simulink model "Simulation_control"  (R2024a)
settings: Solver=ode4  StartTime=0.0  StopTime=105  FixedStep=0.01  RelTol=1e-3
InitFcn:
  | SimInit
values from neighbouring files (symbols this model uses):
  A_mdl = [A11 0 0 ... (first row only)    [SimInit.m]
  B_mdl = l*Kvt/(r*R) * [0 sqrt(3)/(2*M), -sqrt(3)/(2*M) ... (first row only)    [SimInit.m]
  k1_smc = diag([0.7206586704988028 0.846888480151037 0.848909652523])    [SimInit.m]
  k2_smc = diag([1.3 1.32370704517714 1.1]) * k1_smc    [SimInit.m]
  K_mdl = [-Cv/M 0 0 ... (first row only)    [SimInit.m]
  Q_smc = 0.1*diag([1, 1, 1])    [SimInit.m]
settings Model: Creator=irfan  LastModifiedBy=irfan
settings DataIOCC: LimitDataPoints=on  MaxDataPoints=1

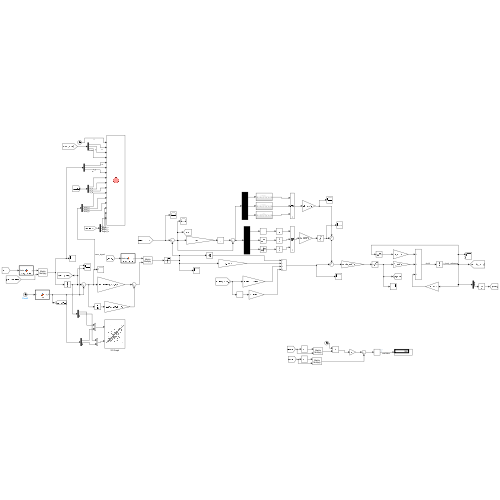
[thumbnail: Simulink's stored preview of the top-level diagram]
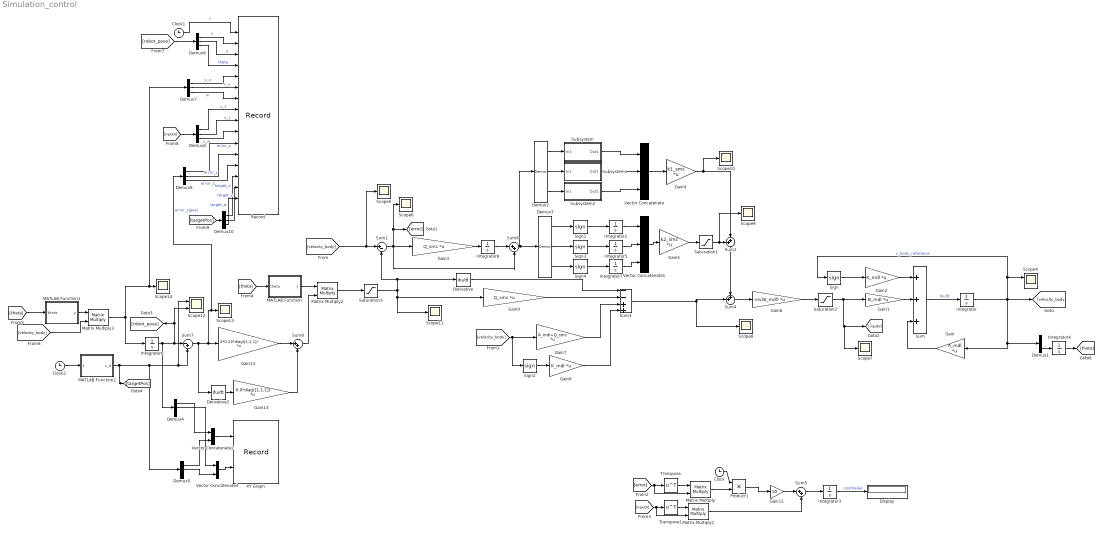
== system Simulation_control ==
  Clock : Clock
  Clock1 : Clock
  Clock2 : Clock
  Demux{1..10} (10 alike) : Demux  Outputs=3
  Derivative : Derivative
  Derivative2 : Derivative
  Display : Display
  Gain : Gain  Gain=A_mdl  Multiplication=Matrix(K*u)
  Gain1 : Gain  Gain=B_mdl  Multiplication=Matrix(K*u)
  Gain11 : Gain  Gain=10
  Gain13 : Gain  Gain=4*0.23*diag([1,1,1])  Multiplication=Matrix(K*u)
  Gain14 : Gain  Gain=0.9*diag([1,1,1])  Multiplication=Matrix(K*u)
  Gain2 : Gain  Gain=K_mdl  Multiplication=Matrix(K*u)
  Gain3 : Gain  Gain=Q_smc  Multiplication=Matrix(K*u)
  Gain4 : Gain  Gain=k1_smc  Multiplication=Matrix(K*u)
  Gain5 : Gain  Gain=k2_smc  Multiplication=Matrix(K*u)
  Gain6 : Gain  Gain=-inv(B_mdl)  Multiplication=Matrix(K*u)
  Gain7 : Gain  Gain=A_mdl+Q_smc  Multiplication=Matrix(K*u)
  Gain8 : Gain  Gain=K_mdl  Multiplication=Matrix(K*u)
  Gain9 : Gain  Gain=Q_smc  Multiplication=Matrix(K*u)
  Integrator{,2..5,7..8} (7 alike) : Integrator
  Integrator6 : Integrator  InitialCondition=[2;-1;0]
  MATLAB Function : MATLAB Function  TreatAsAtomicUnit=on
  MATLAB Function1 : MATLAB Function  TreatAsAtomicUnit=on
  MATLAB Function2 : MATLAB Function  TreatAsAtomicUnit=on
  Matrix Multiply{,1..3} (4 alike) : Product  Multiplication=Matrix(*)
  Product1 : Product
  Record : Record  Filename=result_10kg.mat  RecordToFile=on  FileSettingsInternal="{\"entries\":[{\"content\":{\"excelSettings\":{\"content\":{},\"type\":\"Streamout.ExcelSettings\"}},\"type\":\"Streamout.FileSettingStorage\",\"uuid\":\"\"}],\"packageUris\":[\"http:\\/\\/schema.mathworks.com\\/mf0\\/streamout_blocks\\/R2020a\"],\"version\":\"1.0\"}"  SignalsInternal="{\"entries\":[{\"content\":{\"signals\":[{\"content\":{\"blockPath\":[],\"dimensions\":[1],\"domain\":\"\",\"lineColor\":\"#64d413\",\"lineWidth\":2,\"plots\":[ 1 ],\"port\":1,\"sid\":[\"\"],\"signalID\":1,\"signalName\":\"t\"},\"type\":\"RecordBlkView.Signal\",\"uuid\":\"\"},{\"content\":{\"blockPath\":[],\"dimensions\":[1,1],\"domain\":\"\",\"lineColor\":\"#ff13a6\",\"lineWidth\":2,\"plots\":[ 1 ],\"port\":2,\"sid\":[\"\"],\"signalID\":2,\"signalName\":\"x\"},\"type\":\"RecordBlkView.Signal\",\"uuid\":\"\"},{\"content\":{\"blockPath\":[],\"dimensions\":[1,1],\"domain\":\"\",\"lineColor\":\"#fe330a\",\"lineWidth\":2,\"plots\":[ 1 ],\"port\":3,\"sid\":[\"\"],\"signalID\":3,\"signalName\":\"y\"},\"type\":\"RecordBlkView.Signal\",\"uuid\":\"\"},{\"content\":{\"blockPath\":[],\"dimensions\":[1,1],\"domain\":\"\",\"lineColor\":\"#22b573\",\"lineWidth\":2,\"plots\":[ 1 ],\"port\":4,\"sid\":[\"\"],\"signalID\":4,\"signalName\":\"theta\"},\"type\":\"RecordBlkView.Signal\",\"uuid\":\"\"},{\"content\":{\"blockPath\":[],\"dimensions\":[1,1],\"domain\":\"\",\"lineColor\":\"#0072bd\",\"lineWidth\":2,\"plots\":[ 1 ],\"port\":5,\"sid\":[\"\"],\"signalID\":5,\"signalName\":\"v_x\"},\"type\":\"RecordBlkView.Signal\",\"uuid\":\"\"},{\"content\":{\"blockPath\":[],\"dimensions\":[1,1],\"domain\":\"\",\"lineColor\":\"#d95319\",\"lineWidth\":2,\"plots\":[ 1 ],\"port\":6,\"sid\":[\"\"],\"signalID\":6,\"signalName\":\"v_y\"},\"type\":\"RecordBlkView.Signal\",\"uuid\":\"\"},{\"content\":{\"blockPath\":[],\"dimensions\":[1,1],\"domain\":\"\",\"lineColor\":\"#edb120\",\"lineWidth\":2,\"plots\":[ 1 ],\"port\":7,\"sid\":[\"\"],\"signalID\":7,\"signalName\":\"w\"},\"type\":\"RecordBlkView.Signal\",\"uuid\":\"\"},{\"content\":{\"blockPath\":[],\"dimensions\":[1,1],\"domain\":\"\",\"lineColor\":\"#a2142f\",\"lineWidth\":2,\"plots\":[ 1 ],\"port\":8,\"sid\":[\"\"],\"signalID\":8,\"signalName\":\"u_x\"},\"type\":\"RecordBlkView.Signal\",\"uuid\":\"\"},{\"content\":{\"blockPath\":[],\"dimensions\":[1,1],\"domain\":\"\",\"lineColor\":\"#139fff\",\"lineWidth\":2,\"plots\":[ 1 ],\"port\":9,\"sid\":[\"\"],\"signalID\":9,\"signalName\":\"u_y\"},\"type\":\"RecordBlkView.Signal\",\"uuid\":\"\"},{\"content\":{\"blockPath\":[],\"dimensions\":[1,1],\"domain\":\"\",\"lineColor\":\"#ff6929\",\"lineWidth\":2,\"plots\":[ 1 ],\"port\":10,\"sid\":[\"\"],\"signalID\":10,\"signalName\":\"u_w\"},\"type\":\"RecordBlkView.Signal\",\"uuid\":\"\"},{\"content\":{\"blockPath\":[],\"dimensions\":[1,1],\"domain\":\"\",\"lineColor\":\"#b746ff\",\"lineWidth\":2,\"plots\":[ 1 ],\"port\":11,\"sid\":[\"\"],\"signalID\":11,\"signalName\":\"error_x\"},\"type\":\"RecordBlkView.Signal\",\"uuid\":\"\"},{\"content\":{\"blockPath\":[],\"dimensions\":[1,1],\"domain\":\"\",\"lineColor\":\"#64d413\",\"lineWidth\":2,\"plots\":[ 1 ],\"port\":12,\"sid\":[\"\"],\"signalID\":12,\"signalName\":\"error_y\"},\"type\":\"RecordBlkView.Signal\",\"uuid\":\"\"},{\"content\":{\"blockPath\":[],\"dimensions\":[1,1],\"domain\":\"\",\"lineColor\":\"#ff13a6\",\"lineWidth\":2,\"plots\":[ 1 ],\"port\":13,\"sid\":[\"\"],\"signalID\":13,\"signalName\":\"error_z\"},\"type\":\"RecordBlkView.Signal\",\"uuid\":\"\"},{\"content\":{\"blockPath\":[],\"dimensions\":[1,1],\"domain\":\"\",\"lineColor\":\"#77ac30\",\"lineWidth\":2,\"plots\":[ 1 ],\"port\":14,\"sid\":[\"\"],\"signalID\":14,\"signalName\":\"target_x\"},\"type\":\"RecordBlkView.Signal\",\"uuid\":\"\"},{\"content\":{\"blockPath\":[],\"dimensions\":[1,1],\"domain\":\"\",\"lineColor\":\"#4dbeee\",\"lineWidth\":2,\"plots\":[ 1 ],\"port\":15,\"sid\":[\"\"],\"signalID\":15,\"signalName\":\"target_y\"},\"type\":\"RecordBlkView.Signal\",\"uuid\":\"\"},{\"content\":{\"blockPath\":[],\"dimensions\":[1,1],\"domain\":\"\",\"lineColor\":\"#a2142f\",\"lineWidth\":2,\"plots\":[ 1 ],\"port\":16,\"sid\":[\"\"],\"signalID\":16,\"signalName\":\"target_w\"},\"type\":\"RecordBlkView.Signal\",\"uuid\":\"\"}]},\"type\":\"RecordBlkView.InputSignals\",\"uuid\":\"\"}],\"packageUris\":[\"http:\\/\\/schema.mathworks.com\\/mf0\\/streamout_blocks\\/R2020a\"],\"version\":\"1.0\"}"  VisualizationBindings="{\"sparklinesplugin\":{\"info\":[{\"bindingParametersList\":[],\"subplotID\":1}]}}"
  Saturation1 : Saturate  UpperLimit=12  LowerLimit=-12
  Saturation2 : Saturate  UpperLimit=6  LowerLimit=-6
  Saturation3 : Saturate  UpperLimit=[2.3;2.3;28]  LowerLimit=-[2.3;2.3;28]
  Scope{5..11,13..14} (9 alike) : Scope
  Scope12 : Scope  NumInputPorts=2
  Scope4 : Scope  NumInputPorts=2
  Sign{,1..4} (5 alike) : Signum
  Subsystem : Subsystem
  Subsystem1 : Subsystem
  Subsystem2 : Subsystem
  Sum : Sum  Inputs=+++
  Sum1 : Sum  Inputs=|+-
  Sum2 : Sum  Inputs=++|
  Sum3 : Sum  Inputs=--++
  Sum4 : Sum  Inputs=++|
  Sum5 : Sum  Inputs=|++
  Sum6 : Sum  Inputs=|++
  Sum7 : Sum  Inputs=|-+
  Sum8 : Sum  Inputs=|++
  Transpose : Math  Operator=transpose
  Transpose1 : Math  Operator=transpose
  Vector Concatenate : Concatenate  NumInputs=3  Mode=Multidimensional array
  Vector Concatenate1 : Concatenate  NumInputs=3  Mode=Multidimensional array
  Vector Concatenate2 : Concatenate  Mode=Multidimensional array
  Vector Concatenate3 : Concatenate  Mode=Multidimensional array
  XY Graph : Record  Filename=recording.mat  RecordToFile=on  FileSettingsInternal="{\"entries\":[{\"content\":{\"excelSettings\":{\"content\":{},\"type\":\"Streamout.ExcelSettings\"}},\"type\":\"Streamout.FileSettingStorage\",\"uuid\":\"\"}],\"packageUris\":[\"http:\\/\\/schema.mathworks.com\\/mf0\\/streamout_blocks\\/R2020a\"],\"version\":\"1.0\"}"  Layout=[1 1]  SignalsInternal="{\"entries\":[{\"content\":{\"signals\":[{\"content\":{\"blockPath\":[],\"dimensions\":[2,1],\"domain\":\"\",\"hasChildren\":true,\"lineColor\":\"#ff6929\",\"lineWidth\":2,\"port\":1,\"sid\":[\"\"],\"signalID\":1,\"signalName\":\"Vector\\nConcatenate2\"},\"type\":\"RecordBlkView.Signal\",\"uuid\":\"\"},{\"content\":{\"blockPath\":[],\"channel\":[1,1],\"dimensions\":[2,1],\"domain\":\"\",\"lineColor\":\"#edb120\",\"lineWidth\":2,\"parentID\":1,\"plots\":[ 1 ],\"port\":1,\"sid\":[\"\"],\"signalID\":2,\"signalName\":\"Vector\\nConcatenate2\"},\"type\":\"RecordBlkView.Signal\",\"uuid\":\"\"},{\"content\":{\"blockPath\":[],\"dimensions\":[2,1],\"domain\":\"\",\"hasChildren\":true,\"lineColor\":\"#64d413\",\"lineWidth\":2,\"port\":2,\"sid\":[\"\"],\"signalID\":3,\"signalName\":\"Vector\\nConcatenate3\"},\"type\":\"RecordBlkView.Signal\",\"uuid\":\"\"},{\"content\":{\"blockPath\":[],\"channel\":[1,1],\"dimensions\":[2,1],\"domain\":\"\",\"lineColor\":\"#77ac30\",\"lineWidth\":2,\"parentID\":3,\"plots\":[ 1 ],\"port\":2,\"sid\":[\"\"],\"signalID\":4,\"signalName\":\"Vector\\nConcatenate3\"},\"type\":\"RecordBlkView.Signal\",\"uuid\":\"\"},{\"content\":{\"blockPath\":[],\"channel\":[2,1],\"dimensions\":[2,1],\"domain\":\"\",\"lineColor\":\"#4dbeee\",\"lineWidth\":2,\"parentID\":1,\"plots\":[ 1 ],\"port\":1,\"sid\":[\"\"],\"signalID\":5,\"signalName\":\"Vector\\nConcatenate2\"},\"type\":\"RecordBlkView.Signal\",\"uuid\":\"\"},{\"content\":{\"blockPath\":[],\"channel\":[2,1],\"dimensions\":[2,1],\"domain\":\"\",\"lineColor\":\"#a2142f\",\"lineWidth\":2,\"parentID\":3,\"plots\":[ 1 ],\"port\":2,\"sid\":[\"\"],\"signalID\":6,\"signalName\":\"Vector\\nConcatenate3\"},\"type\":\"RecordBlkView.Signal\",\"uuid\":\"\"}]},\"type\":\"RecordBlkView.InputSignals\",\"uuid\":\"\"}],\"packageUris\":[\"http:\\/\\/schema.mathworks.com\\/mf0\\/streamout_blocks\\/R2020a\"],\"version\":\"1.0\"}"  VisualizationBindings="{\"xyplotplugin\":{\"info\":[{\"series\":[{\"bindingParametersList\":[{\"parameter\":\"X-Axis\",\"signalID\":2,\"signalName\":\"Vector\\nConcatenate2(1,1)\"},{\"parameter\":\"Y-Axis\",\"signalID\":4,\"signalName\":\"Vector\\nConcatenate3(1,1)\"}],\"seriesID\":0},{\"bindingParametersList\":[{\"parameter\":\"X-Axis\",\"signalID\":5,\"signalName\":\"Vector\\nConcatenate2(2,1)\"},{\"parameter\":\"Y-Axis\",\"signalID\":6,\"signalName\":\"Vector\\nConcatenate3(2,1)\"}],\"seriesID\":1}],\"subplotID\":1}]}}"  CompatibilityTag=XY
  wires:
  Sum/1 -> Integrator/1  "dv/dt"
  Integrator/1 -> Sign/1, Scope4/1, [velocity_body], Demux1/1, Gain/1  "v_body_reference"
  Gain/1 -> Sum/3
  Gain1/1 -> Sum/2
  Gain2/1 -> Sum/1
  Sign/1 -> Gain2/1
  Demux1/3 -> Integrator4/1
  Integrator4/1 -> [theta]
  [velocity_body] -> Scope5/1, Sum1/1
  [velocity_body] -> Sign2/1, Gain7/1
  Sign2/1 -> Gain8/1
  Gain7/1 -> Sum3/3
  Gain8/1 -> Sum3/4
  [error] -> Matrix Multiply/2, Transpose/1
  Transpose/1 -> Matrix Multiply/1
  Matrix Multiply/1 -> Product1/2
  Gain11/1 -> Sum5/1
  [inputU] -> Matrix Multiply1/2, Transpose1/1
  Transpose1/1 -> Matrix Multiply1/1
  Matrix Multiply1/1 -> Sum5/2
  Clock/1 -> Product1/1
  Product1/1 -> Gain11/1
  Integrator3/1 -> Display/1  "costValue"
  Sum5/1 -> Integrator3/1
  Sum4/1 -> Gain6/1
  [theta] -> MATLAB Function/1(theta)
  MATLAB Function/1(y) -> Matrix Multiply2/1
  [theta] -> MATLAB Function1/1(theta)
  MATLAB Function1/1(y) -> Matrix Multiply3/1
  [velocity_body] -> Matrix Multiply3/2
  Matrix Multiply3/1 -> Integrator6/1, Demux7/1, Scope14/1
  Integrator6/1 -> Demux4/1, Scope12/2, [robot_pose], Sum7/1
  MATLAB Function2/1(x_d) -> [targetPos], Demux5/1, Scope12/1, Sum7/2
  Sum7/1 -> Demux9/1, Scope13/1, Gain13/1, Derivative2/1  "error_signal"
  Gain13/1 -> Sum8/1
  Derivative2/1 -> Gain14/1
  Gain14/1 -> Sum8/2
  Sum8/1 -> Matrix Multiply2/2
  Matrix Multiply2/1 -> Saturation3/1
  Demux2/1 -> Subsystem/1(In1)
  Demux2/2 -> Subsystem1/1(In1)
  Demux2/3 -> Subsystem2/1(In1)
  Subsystem/1(Out1) -> Vector Concatenate/1
  Subsystem1/1(Out1) -> Vector Concatenate/2
  Subsystem2/1(Out1) -> Vector Concatenate/3
  Vector Concatenate/1 -> Gain4/1
  Demux3/1 -> Sign1/1
  Demux3/2 -> Sign3/1
  Demux3/3 -> Sign4/1
  Sign1/1 -> Integrator2/1
  Sign3/1 -> Integrator5/1
  Sign4/1 -> Integrator7/1
  Integrator2/1 -> Vector Concatenate1/1
  Integrator5/1 -> Vector Concatenate1/2
  Integrator7/1 -> Vector Concatenate1/3
  Vector Concatenate1/1 -> Gain5/1
  Gain4/1 -> Scope10/1, Sum2/2
  Sum2/1 -> Sum4/1
  Sum3/1 -> Sum4/2, Scope8/1
  Gain5/1 -> Saturation1/1
  Saturation3/1 -> Derivative/1, Sum1/2, Gain9/1, Scope11/1
  Gain6/1 -> Saturation2/1
  Saturation1/1 -> Scope9/1, Sum2/1
  Vector Concatenate2/1 -> XY Graph/1
  Demux4/1 -> Vector Concatenate2/1
  Demux5/1 -> Vector Concatenate2/2
  Vector Concatenate3/1 -> XY Graph/2
  Demux4/2 -> Vector Concatenate3/1
  Demux5/2 -> Vector Concatenate3/2
  Saturation2/1 -> Gain1/1, Scope7/1, [inputU]
  Clock1/1 -> Record/1  "t"
  [robot_pose] -> Demux6/1
  Demux6/1 -> Record/2  "x"
  Demux6/2 -> Record/3  "y"
  Demux6/3 -> Record/4  "theta"
  Demux7/1 -> Record/5  "v_x"
  Demux7/2 -> Record/6  "v_y"
  Demux7/3 -> Record/7  "w"
  Clock2/1 -> MATLAB Function2/1(t)
  Sum6/1 -> Demux2/1, Demux3/1
  Integrator8/1 -> Sum6/1
  Sum1/1 -> Sum6/2, Gain3/1, Scope6/1, [error]
  Gain3/1 -> Integrator8/1
  Gain9/1 -> Sum3/2
  Derivative/1 -> Sum3/1
  [inputU] -> Demux8/1
  Demux8/1 -> Record/8  "u_x"
  Demux8/2 -> Record/9  "u_y"
  Demux8/3 -> Record/10  "u_w"
  Demux9/1 -> Record/11  "error_x"
  Demux9/2 -> Record/12  "error_y"
  Demux9/3 -> Record/13  "error_z"
  [targetPos] -> Demux10/1
  Demux10/1 -> Record/14  "target_x"
  Demux10/2 -> Record/15  "target_y"
  Demux10/3 -> Record/16  "target_w"

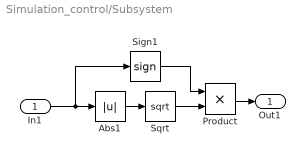
== system Simulation_control/Subsystem ==
  In1 : Inport
  Abs1 : Abs  SaturateOnIntegerOverflow=off
  Product : Product
  Sign1 : Signum
  Sqrt : Sqrt
  Out1 : Outport
  wires:
  Sqrt/1 -> Product/2
  In1/1 -> Sign1/1, Abs1/1
  Abs1/1 -> Sqrt/1
  Sign1/1 -> Product/1
  Product/1 -> Out1/1

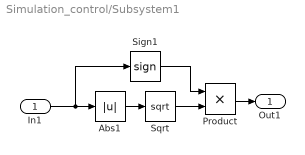
== system Simulation_control/Subsystem1 ==
  In1 : Inport
  Abs1 : Abs  SaturateOnIntegerOverflow=off
  Product : Product
  Sign1 : Signum
  Sqrt : Sqrt
  Out1 : Outport
  wires:
  Product/1 -> Out1/1
  Sign1/1 -> Product/1
  Abs1/1 -> Sqrt/1
  In1/1 -> Abs1/1, Sign1/1
  Sqrt/1 -> Product/2

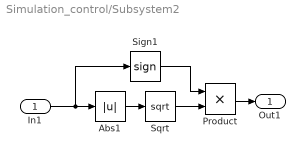
== system Simulation_control/Subsystem2 ==
  In1 : Inport
  Abs1 : Abs  SaturateOnIntegerOverflow=off
  Product : Product
  Sign1 : Signum
  Sqrt : Sqrt
  Out1 : Outport
  wires:
  Sqrt/1 -> Product/2
  In1/1 -> Sign1/1, Abs1/1
  Abs1/1 -> Sqrt/1
  Sign1/1 -> Product/1
  Product/1 -> Out1/1

== matlab function Simulation_control/MATLAB Function1 ==
  data: theta input; y output
function y = body2world(theta)

y = [cos(theta), -sin(theta), 0;
     sin(theta), cos(theta), 0;
     0, 0, 1];

== matlab function Simulation_control/MATLAB Function2 ==
  data: t input; x_d output
function x_d = fcn(t)
T = 100;
if t <= T/4
    x_d = [10 * t / (T/4); 0; 0];  % Move along x-axis
elseif t <= T/2
    x_d = [10; 5 * (t - T/4) / (T/4); 0];  % Move along y-axis
elseif t <= 3*T/4
    x_d = [10 - 10 * (t - T/2) / (T/4); 5; 0];  % Move back along x-axis
elseif t <= T
    x_d = [0; 5 - 5 * (t - 3*T/4) / (T/4); 0];  % Move back along y-axis
else
    x_d = [0;0;0];
end

== matlab function Simulation_control/MATLAB Function ==
  data: theta input; y output
function y = world2body(theta)

y = [cos(theta), -sin(theta), 0;
     sin(theta), cos(theta), 0;
     0, 0, 1]';
